simulink model "Question_3"  (R2024b)
settings: Solver=VariableStepAuto  StartTime=0.0  StopTime=10.0  RelTol=1e-3
model workspace (MAT data in the model file):
  M = 100
  b = 0.5
  k = 1
settings Model: Creator=Sagar  LastModifiedBy=Sagar

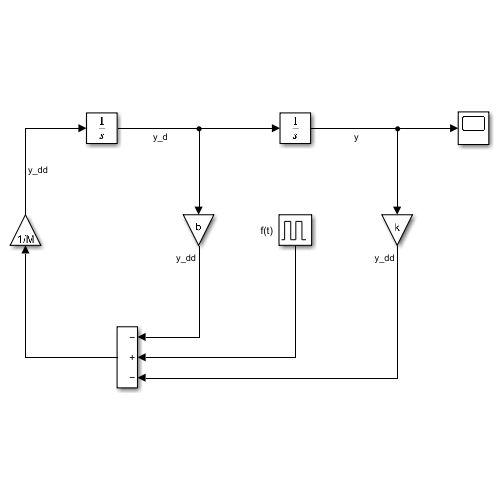
[thumbnail: Simulink's stored preview of the top-level diagram]
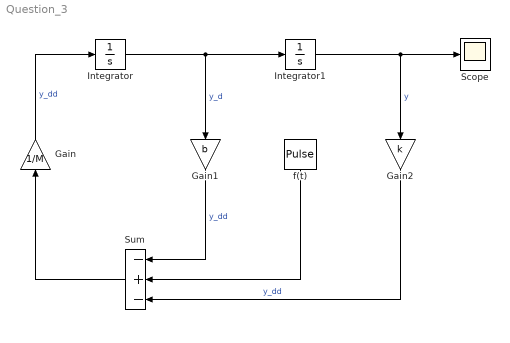
== system Question_3 ==
  Gain : Gain  Gain=1/M
  Gain1 : Gain  Gain=b
  Gain2 : Gain  Gain=k
  Integrator : Integrator
  Integrator1 : Integrator  InitialCondition=1.8
  Scope : Scope
  Sum : Sum  Inputs=-+-
  f(t) : DiscretePulseGenerator  PulseType=Time based  Period=10  PulseWidth=5
  wires:
  Integrator/1 -> Gain1/1, Integrator1/1  "y_d"
  Gain/1 -> Integrator/1  "y_dd"
  Integrator1/1 -> Scope/1, Gain2/1  "y"
  f(t)/1 -> Sum/2
  Gain1/1 -> Sum/1  "y_dd"
  Gain2/1 -> Sum/3  "y_dd"
  Sum/1 -> Gain/1
